simulink model "FSK"  (R2017a)
settings: Solver=VariableStepAuto  StartTime=0.0  StopTime=10000  RelTol=1e-3
libraries: commdigbbndfm2 x2, commchan3 x1, commsink2 x1, commrandsrc3 x1
settings Model: Creator=AmmarRabie  LastModifiedBy=AmmarRabie

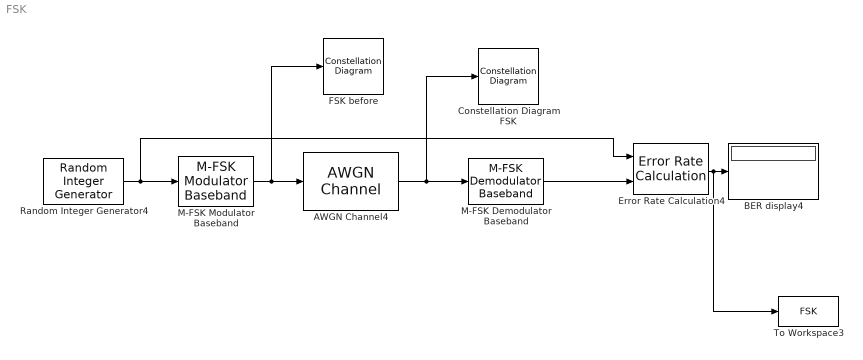
== system FSK ==
  AWGN Channel4 : commchan3/AWGN Channel  InputProcessing=Columns as channels (frame based)  seed=67  noiseMode="Signal to noise ratio  (Eb/No)"  EbNodB=EbNo  EsNodB=10  SNRdB=10  bitsPerSym=1  Ps=1  Tsym=1  variance=1
  BER display4 : Display
  Constellation Diagram FSK : ConstellationDiagram
  Error Rate Calculation4 : commsink2/Error Rate Calculation  N=0  st_delay=0  cp_mode=Entire frame  subframe=[]  PMode=Port  WsName=ErrorVec  RsMode2=off  stop=off  numErr=100  maxBits=1e6
  FSK before : ConstellationDiagram
  M-FSK Demodulator Baseband : commdigbbndfm2/M-FSK Demodulator Baseband  M=2  OutType=Integer  Dec=Gray  freqSep=6  numSamp=17  RateOptions=Enforce single-rate processing  outDataType=double
      settings: SourceProductName=Communications System Toolbox  SourceProductBaseCode=CM
  M-FSK Modulator Baseband : commdigbbndfm2/M-FSK Modulator Baseband  M=2  InType=Integer  Enc=Gray  freqSep=6  phaseType=Continuous  numSamp=17  RateOptions=Enforce single-rate processing  outDataType=double
      settings: SourceProductName=Communications System Toolbox
  Random Integer Generator4 : commrandsrc3/Random Integer Generator  SetSize=2  SeedSource=Parameter  Seed=37  SampleTime=1  SamplesPerFrame=100  OutputDataType=double  SimulateUsing=Interpreted execution
  To Workspace3 : ToWorkspace  VariableName=FSK  SampleTime=-1
      settings: MaxDataPoints=2  Save2DSignal=2-D array (concatenate along first dimension)
  wires:
  M-FSK Modulator Baseband/1 -> FSK before/1, AWGN Channel4/1
  AWGN Channel4/1 -> M-FSK Demodulator Baseband/1, Constellation Diagram FSK/1
  Error Rate Calculation4/1 -> To Workspace3/1, BER display4/1
  M-FSK Demodulator Baseband/1 -> Error Rate Calculation4/2
  Random Integer Generator4/1 -> M-FSK Modulator Baseband/1, Error Rate Calculation4/1
